simulink model "untitled"  (R2020a)
settings: Solver=FixedStepAuto  StartTime=0.0  StopTime=inf  FixedStep=0.001  RelTol=1e-3
undefined symbols (not defined in the file): Standard_Devices, UDP_Protocol
libraries: sldrtlib x3
settings Model: Creator=10105  LastModifiedBy=10105

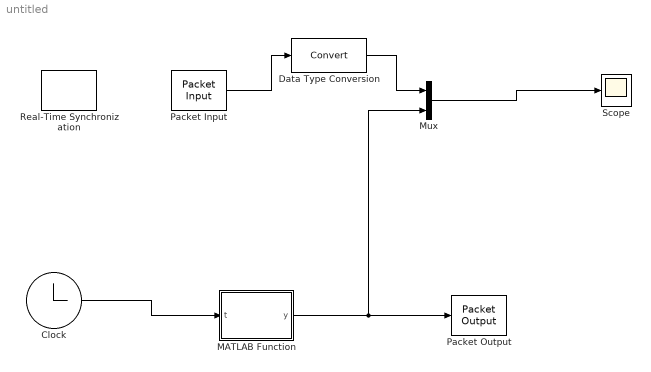
== system untitled ==
  Clock : Clock
  Data Type Conversion : DataTypeConversion
  MATLAB Function : MATLAB Function  TreatAsAtomicUnit=on
  Mux : Mux  Inputs=2
  Packet Input : sldrtlib/Packet Input  SampleTime=-1  MaxMissedTicks=1000000  ShowMissedTicks=off  YieldWhenWaiting=off  DrvName=Standard_Devices/UDP_Protocol  DrvAddress=8888  DrvOptions=[0 8888 49 57 50 46 49 54 56 46 50 48 48 46 51 0 0 0 0 0 0 0 0 0 0 0 0 0 0 0 0 0 0 0 0 0 0 0 0 0 0 0 0 0 0 0 0 0 0 0 0 0 0 0 0 0 0 0 0 0 0 0 0 0 0 0 0 0 0 0 0 0 0 0 0 0 0 0 0 0 0 0 0 0 0 0 0 0 0 0 0 0 0 0 0 0 0 0 0 0 0 0 0 0 0 0 0 0 0 0 0 0 0 0 0 0 0 0 0 0 0 0 0 0 0 0 0 0 0 0 0 0 0 0 0 0 0 0 0 0 0 0 0 0 0 0 0 0 0 0 0 0 0 0 0 0 0 0 0 0 0 0 0 0 0 0 0 0 0 0 0 0 0 0 0 0 0 0 0 0 0 0 0 0 0 0 0 0 0 0 0 0 0 0 0 0 0 0 0 0 0 0 0 0 0 0 0 0 0 0 0 0 0 0 0 0 0 0 0 0 0 0 0 0 0 0 0 0 0 0 0 0 0 0 0 0 0 0 0 0 0 0 0 0 0 0 0 0 0 0 0 0 0 0 0 0]  PacketSize=1  DataTypes='1*uint8'  ShowReady=off  ShowError=off  PacketID=1  ByteOrder=1  ShowTimestamp=off
      settings: AttributesFormatString=UDP Protocol [8888]
  Packet Output : sldrtlib/Packet Output  SampleTime=-1  MaxMissedTicks=1000000  ShowMissedTicks=off  YieldWhenWaiting=off  DrvName=Standard_Devices/UDP_Protocol  DrvAddress=8888  DrvOptions=[0 8888 49 57 50 46 49 54 56 46 50 48 48 46 51 0 0 0 0 0 0 0 0 0 0 0 0 0 0 0 0 0 0 0 0 0 0 0 0 0 0 0 0 0 0 0 0 0 0 0 0 0 0 0 0 0 0 0 0 0 0 0 0 0 0 0 0 0 0 0 0 0 0 0 0 0 0 0 0 0 0 0 0 0 0 0 0 0 0 0 0 0 0 0 0 0 0 0 0 0 0 0 0 0 0 0 0 0 0 0 0 0 0 0 0 0 0 0 0 0 0 0 0 0 0 0 0 0 0 0 0 0 0 0 0 0 0 0 0 0 0 0 0 0 0 0 0 0 0 0 0 0 0 0 0 0 0 0 0 0 0 0 0 0 0 0 0 0 0 0 0 0 0 0 0 0 0 0 0 0 0 0 0 0 0 0 0 0 0 0 0 0 0 0 0 0 0 0 0 0 0 0 0 0 0 0 0 0 0 0 0 0 0 0 0 0 0 0 0 0 0 0 0 0 0 0 0 0 0 0 0 0 0 0 0 0 0 0 0 0 0 0 0 0 0 0 0 0 0 0 0 0 0 0 0 0]  PacketSize=6  DataTypes='6*uint8'  ShowReady=off  ShowError=off  PacketID=1  ByteOrder=1  InitialValue=[]  FinalValue=[]
      settings: AttributesFormatString=UDP Protocol [8888]
  Real-Time Synchronization : sldrtlib/Real-Time Synchronization  SampleTime=0.002  MaxMissedTicks=1000  ShowMissedTicks=off  YieldWhenWaiting=off
  Scope : Scope
  wires:
  Clock/1 -> MATLAB Function/1(t)
  MATLAB Function/1(y) -> Mux/2, Packet Output/1
  Packet Input/1 -> Data Type Conversion/1
  Mux/1 -> Scope/1
  Data Type Conversion/1 -> Mux/1

== matlab function untitled/MATLAB Function ==
  data: t input; y output
function y = fcn(t)
%stepper 1, stepper 2, DC 1, DC 2, DC 3, DC 4. 
% [angular pos1, pos2, pos3, pos4, pos5, pos6]
% % range: 0~255
st1max = 120;
st2max = 170;
dc1max = 120;
dc2max = 180; %90
dc3max = 80; %90
dc4max = 140;
if t < 5
   y = [0, 0, 0, 0, 0, 0];
elseif t < 10
   y = [0, 0, 0, dc2max, 0, 0];
elseif t < 15
   y = [0, 0, 0, dc2max, dc3max, 0];
elseif t < 25
   y = [0, st2max, 0, dc2max, dc3max, 0];
elseif t < 55
   y = [st1max, st2max, 0, dc2max, dc3max, 0];
elseif t < 60
   y = [st1max, st2max, 0, dc2max, dc3max, dc4max];
elseif t < 100
   y = [0, st2max, 0, dc2max, dc3max, dc4max];
elseif t < 105
   y = [0, st2max, dc1max, dc2max, dc3max, dc4max];
elseif t < 110
   y = [0, st2max, dc1max, dc2max, dc3max, 0];
else
   y = [0, st2max, 0, dc2max, dc3max, 0];
end
end

% dc3: 90
% dc4: 140
% if t<5
%     y = [0,0,0,0,0,0];
% elseif t<10
%     y = [0,0,dc1max, 0,0,0];
% else
%     y = [0,0,0,0,0,0];
% end
% end
